simulink model "complex_with_simpower"  (Simulink 8.0)
settings: Solver=ode45  StartTime=0.0  StopTime=10.0  RelTol=1e-3
settings Model: Creator=rstarr  LastModifiedBy=rstarr

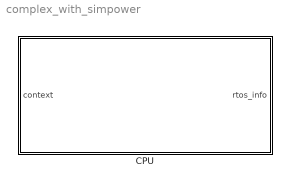
== system complex_with_simpower ==
  CPU : Subsystem  InitFcn=|  mask(Central Processing Unit){custom_block_type=Cpu, slot_number=0, fixed_slot=off, lower_limit_V=16, upper_limit_V=32, availabilityIndex=1, executionIndex=2, contextIndex=3, parameters_type=Sample based, startingup_time=0, housekeeping_time=0, shuttingdown_time=0, schedule_tasks=off, show_sched_tbl=off}
      | % Get Ts parameter                      
      | Ts =compSys.util.getSimulationStepTime(bdroot(gcbh));
      |                                         
      | updateRtosBlk(gcbh);
      mask prompts: custom_block_type "Custom Block Type"; slot_number "Slot Number"; fixed_slot "Fixed Slot"; lower_limit_V "Power Lower Limit (V):"; upper_limit_V "Power Upper Limit (V):"; availabilityIndex "RTOS Availability Index"; executionIndex "RTOS Execution Index"; contextIndex "RTOS Context Index"; parameters_type "Parameters Type:"; startingup_time "Starting Up Time (number of samples)"; housekeeping_time "House Keeping Time (number of samples)"; shuttingdown_time "Shutting Down Time (number of samples)"; schedule_tasks "Schedule Tasks (click for yes)"; show_sched_tbl "Show Scheduling Table (click for yes)"
      mask help: Processor used in an architectural model.
      mask TypeOptions parameters_type: Sample based | Time based
      mask Display: disp('CPU');

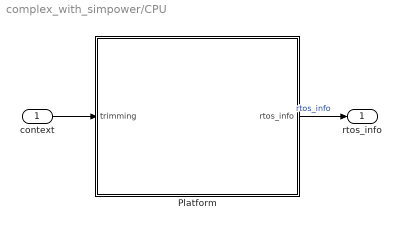
== system complex_with_simpower/CPU ==
  context : Inport
  Platform : Subsystem  Priority=0  mask{custom_block_type=Platform}
      mask prompts: custom_block_type "Custom Block Type"
  rtos_info : Outport
  wires:
  context/1 -> Platform/1(trimming)
  Platform/1(rtos_info) -> rtos_info/1  "rtos_info"

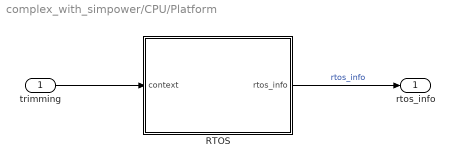
== system complex_with_simpower/CPU/Platform ==
  trimming : Inport
  RTOS : Subsystem  mask{custom_block_type=Rtos, task_quantity=, minor_frame=, minor_frame_info=, minor_frame_quantity=, task_list=, wcetMF=, task_index=}
      mask prompts: custom_block_type "Custom Block Type"; task_quantity "Task Quantity"; minor_frame "Minor Frame (sec)"; minor_frame_info "Minor Frame Information"; minor_frame_quantity "Minor Frame Quantity"; task_list "Task List"; wcetMF "Minor Frame WCET (s)"; task_index "Task Index"
  rtos_info : Outport
  wires:
  trimming/1 -> RTOS/1(context)
  RTOS/1(rtos_info) -> rtos_info/1  "rtos_info"

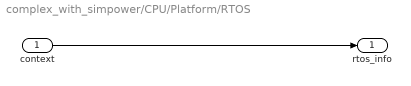
== system complex_with_simpower/CPU/Platform/RTOS ==
  context : Inport
  rtos_info : Outport
  wires:
  context/1 -> rtos_info/1
